simulink subsystem "Circuit_3State_Plant"  (R2022a)
settings: Solver=VariableStepAuto  StartTime=0.0  StopTime=10.0  RelTol=1e-3
values from neighbouring files (symbols this model uses):
  C_des = C    [RunSimulink.m]
  C_m = C_des    [RunSimulink.m]
  K_plant = LC_param.K    [RunSimulink.m]
  M_cross = LC_param.M_cross    [RunSimulink.m]    (also in getLCParam.m = V*S_cross*U')
  SV_IC = SIM.x_0_5    [RunSimulink.m]
  U_NV_NT = LC_param.U_NV_NT    [RunSimulink.m]    (also in getLCParam.m = U_null*V_null')
undefined symbols (not defined in the file or in its folder): A, B, FLAG, N, P, SIM, Ts
settings Model: Creator=tyevans  LastModifiedBy=tyevans

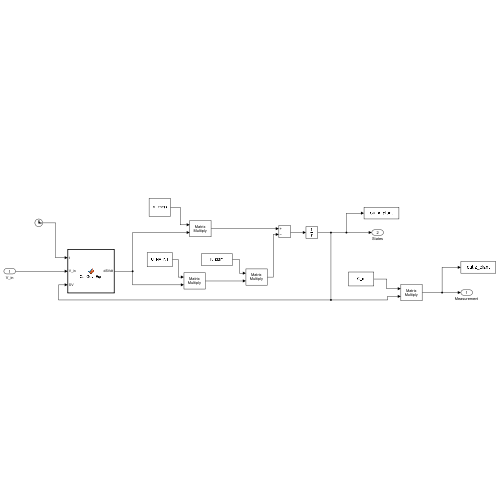
[thumbnail: Simulink's stored preview of the top-level diagram]
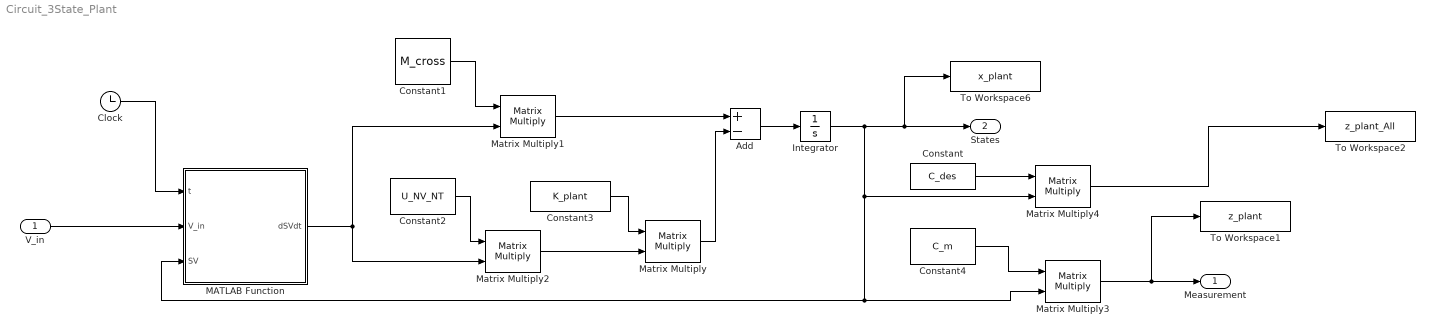
== system Circuit_3State_Plant ==
  V_in : Inport
  Add : Sum  Inputs=+-
  Clock : Clock
  Constant : Constant  Value=C_des  VectorParams1D=off
  Constant1 : Constant  Value=M_cross  VectorParams1D=off
  Constant2 : Constant  Value=U_NV_NT  VectorParams1D=off
  Constant3 : Constant  Value=K_plant  VectorParams1D=off
  Constant4 : Constant  Value=C_m  VectorParams1D=off
  Integrator : Integrator  InitialCondition=SV_IC
  MATLAB Function : MATLAB Function  TreatAsAtomicUnit=on
  Matrix Multiply{,1..4} (5 alike) : Product  Multiplication=Matrix(*)
  To Workspace1 : ToWorkspace  VariableName=z_plant  SaveFormat=Structure With Time  SampleTime=-1
  To Workspace2 : ToWorkspace  VariableName=z_plant_All  SaveFormat=Structure With Time  SampleTime=Ts
  To Workspace6 : ToWorkspace  VariableName=x_plant  SaveFormat=Structure With Time  SampleTime=-1
  Measurement : Outport
  States : Outport  Port=2
  wires:
  Matrix Multiply3/1 -> Measurement/1, To Workspace1/1
  Clock/1 -> MATLAB Function/1(t)
  V_in/1 -> MATLAB Function/2(V_in)
  Constant1/1 -> Matrix Multiply1/1
  Constant2/1 -> Matrix Multiply2/1
  Matrix Multiply1/1 -> Add/1
  Add/1 -> Integrator/1
  Constant4/1 -> Matrix Multiply3/1
  Matrix Multiply/1 -> Add/2
  Constant3/1 -> Matrix Multiply/1
  MATLAB Function/1(dSVdt) -> Matrix Multiply1/2, Matrix Multiply2/2
  Matrix Multiply2/1 -> Matrix Multiply/2
  Constant/1 -> Matrix Multiply4/1
  Matrix Multiply4/1 -> To Workspace2/1
  Integrator/1 -> To Workspace6/1, States/1, MATLAB Function/3(SV), Matrix Multiply3/2, Matrix Multiply4/2

== matlab function Circuit_3State_Plant/MATLAB Function ==
  data: t input; dSVdt output; V_in input; SV input; SIM parameter; N parameter; P parameter; FLAG parameter; A parameter; B parameter
function dSVdt = CallGovnEqn(t,V_in, SV,SIM, N, P, FLAG,A, B)
% Initialize Output
dSVdt = zeros(N.states,1);

% Call Governing Equations
[dSVdt] = GovnEqn_3(t,SV,SIM,N,P,FLAG,A,B,V_in);
end
